simulink model "thrustflapping"  (Simulink 7.7)
settings: Solver=ode45  StartTime=0.0  StopTime=3  RelTol=1e-3
settings Model: Creator=Administrator  LastModifiedBy=Administrator
settings DataIOCC: LimitDataPoints=off  OutputSaveName=T_MR

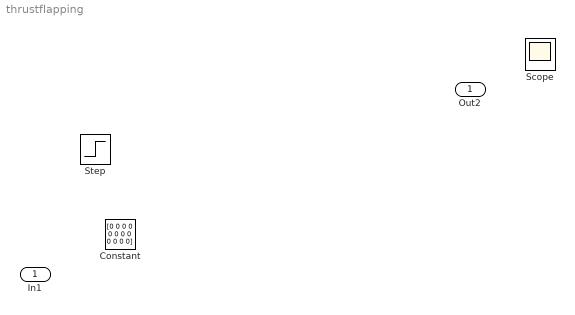
== system thrustflapping ==
  In1 : Inport
  Constant : Constant  Value=[0 0 0 0 0 0 0 0 0 0 0 0]
  Scope : Scope
  Step : Step  Time=0  After=0  SampleTime=0
  Out2 : Outport
  wires:
  ? -> ?
